simulink model "System_Draft"  (R2018b)
settings: Solver=VariableStepAuto  StartTime=0.0  StopTime=10.0  RelTol=1e-3
settings Model: Creator=Whtest  LastModifiedBy=Whtest

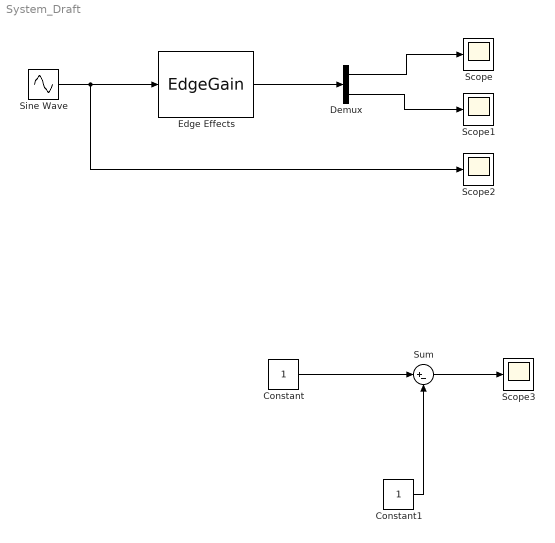
== system System_Draft ==
  Constant : Constant
  Constant1 : Constant
  Demux : Demux  Outputs=2
  Edge Effects : S-Function  FunctionName=EdgeGain  SFunctionDeploymentMode=off  EnableBusSupport=off
  Scope{,1..3} (4 alike) : Scope
  Sine Wave : Sin  Amplitude=1000  Frequency=6.18  SampleTime=0
  Sum : Sum  Inputs=|+-
  wires:
  Demux/2 -> Scope1/1
  Edge Effects/1 -> Demux/1
  Demux/1 -> Scope/1
  Sine Wave/1 -> Scope2/1, Edge Effects/1
  Sum/1 -> Scope3/1
  Constant1/1 -> Sum/2
  Constant/1 -> Sum/1
